simulink library "Lib_Turbo_Compressor_TMATS"  (R2012b)
settings: Solver=ode45  StartTime=0.0  StopTime=10.0  RelTol=1e-3
Description:
  | Thomas Modules
settings Model: Creator=jwchapm2  LastModifiedBy=jwchapm2

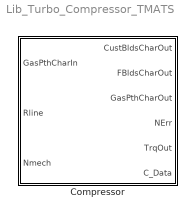
== system Lib_Turbo_Compressor_TMATS ==
  Compressor : Subsystem  mask(T-MATS: Compressor Library Block){X_C_RlineVec_M=[1.000 3.000 ], Y_C_NcVec_M=[0.500  0.900  1.050], T_C_Map_WcArray_M=[0 0; 0 0; 0 0], T_C_Map_PRArray_M=[0 0; 0 0; 0 0], T_C_Map_EffArray_M=[0 0; 0 0; 0 0], s_C_Nc_M=0.0001, s_C_Wc_M=0.4953, s_C_PR_M=0.8636, s_C_Eff_M=0.9977, CBLDEN_M=off, C_CBD_M=0, C_CBFht_M=0.5, C_CBFPt_M=0.5, FBLDEN_M=off, C_FBD_M=0, C_BFht_M=0.5, C_BFPt_M=0.5, X_C_WcSurgeVec_M=[0 200], T_C_PRSurgeVec_M=[30 30], iDesign_M=off, NcDes_M=10000, EffDes_M=0.95, PRDes_M=20, RlineDes_M=2}
      mask prompts: X_C_RlineVec_M "X_C_RlineVec_M - Compressor Map Rline Vector (X-axis)(nx1)"; Y_C_NcVec_M "Y_C_NcVec_M - Compressor Map Corrected Speed Vector (Y-axis)(mx1)"; T_C_Map_WcArray_M "T_C_Map_WcArray_M - Compressor Map Flow Array (Wc = f(Nc, Rline))(mxn)"; T_C_Map_PRArray_M "T_C_Map_PRArray_M - Compressor Map Pressure Ratio Array (PR = f(Nc, Rline))(mxn)"; T_C_Map_EffArray_M "T_C_Map_EffArray_M - Compressor Map Efficiency Array (Eff = f(Nc, Rline)(mxn)"; s_C_Nc_M "s_C_Nc_M - Corrected Speed Scalar Constant (C_Nc)"; s_C_Wc_M "s_C_Wc_M - Flow Scalar Constant (C_Wc)"; s_C_PR_M "s_C_PR_M - Pressure Ratio Scalar Constant (C_PR)"; s_C_Eff_M "s_C_Eff_M - Efficiency Scalar Constant (C_Eff)"; CBLDEN_M "CBLDEN_M - Customer Bleed Enable [0 - off, 1 - on]"; C_CBD_M "C_CBD_M - Customer or flow based Bleed Demand[pps] (cbx1)"; C_CBFht_M "C_CBFht_M - Customer or flow based Bleed Fractional enthalpy[frac] (cbx1)"; C_CBFPt_M "C_CBFPt_M - Customer or flow based Bleed Fractional Total Pressure[frac] (cbx1)"; FBLDEN_M "FBLDEN_M - Customer Bleed Enable [0 - off, 1 - on]"; C_FBD_M "C_FBD_M - Fractional Bleed Demand[frac] (bx1)"; C_BFht_M "C_BFht_M - engine Bleed Fractional enthalpy[frac] (bx1)"; C_BFPt_M "C_BFPt_M - engine Bleed Fractional Total Pressure[frac] (bx1)"; X_C_WcSurgeVec_M "X_C_WcSurgeVec_M - compensated flow Surge vector (sx1)"; T_C_PRSurgeVec_M "T_C_PRSurgeVec_M - Surge Line Pressure Ratio vector (sx1)"; iDesign_M "iDesign_M - Calculate compressor map scalars based on design variables"; NcDes_M "NcDes_M - map Design Corrected Shaft Speed [rpm]"; EffDes_M "EffDes_M  - Design Efficiency [frac]"; PRDes_M "PRDes_M - Design Pressure Ratio [frac]"; RlineDes_M "RlineDes_M - map Design Rline"
      mask help: This block simulates the performance of a compressor using basic thermodynamic equations, properties, and table lookups.
      mask Help: web(which('Turbo_TMATS_Cmp.html'),'-helpbrowser')
      mask Callback CBLDEN_M: MSK_SEC_Enables_TMATS('CBLDEN_M',[11 12 13],'en')
      mask Callback FBLDEN_M: MSK_SEC_Enables_TMATS('FBLDEN_M',[15 16 17],'en')
      mask Callback iDesign_M:
      | MSK_SEC_Enables_TMATS('iDesign_M',[21 22 23 24],'en')
      | MSK_SEC_Enables_TMATS('iDesign_M',[6 7 8 9],'dis')

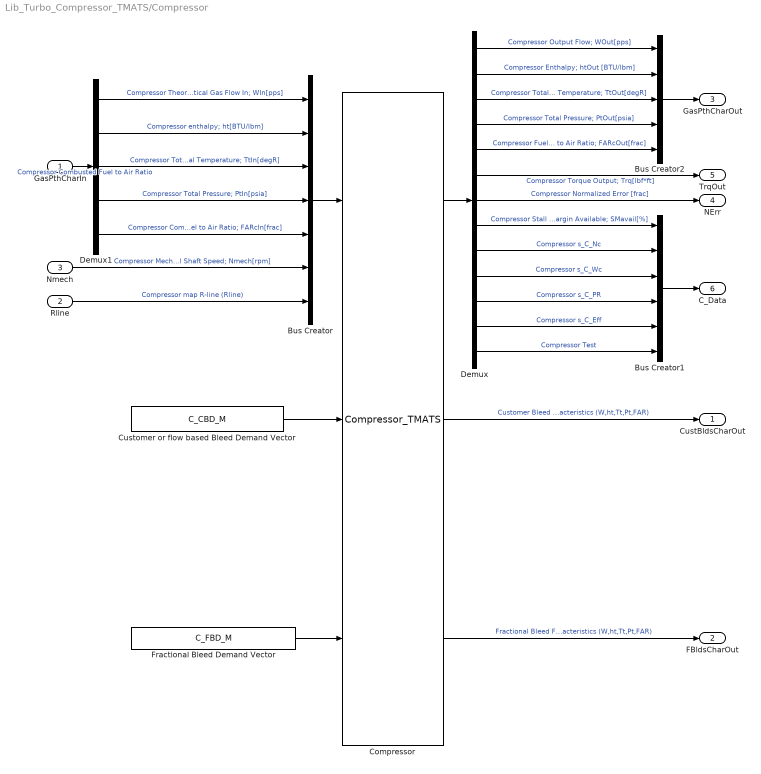
== system Lib_Turbo_Compressor_TMATS/Compressor ==
  GasPthCharIn : Inport
  Rline : Inport  Port=2
  Nmech : Inport  Port=3
  Bus Creator : BusCreator  Inputs=7
  Bus Creator1 : BusCreator  Inputs=6
  Bus Creator2 : BusCreator  Inputs=5
  Compressor : S-Function  FunctionName=Compressor_TMATS  Parameters="s_C_Nc_M, s_C_Wc_M, s_C_PR_M, s_C_Eff_M, Y_C_NcVec_M, X_C_RlineVec_M, T_C_Map_WcArray_M, T_C_Map_PRArray_M, T_C_Map_EffArray_M, C_CBFht_M, C_CBFPt_M,  C_BFht_M, C_BFPt_M, X_C_WcSurgeVec_M, T_C_PRSurgeVec_M, iDesign_M, NcDes_M, EffDes_M, PRDes_M, RlineDes_M, CBLDEN_M, FBLDEN_M, gcs"  EnableBusSupport=off
  Customer or flow based Bleed Demand Vector : Constant  Value=C_CBD_M
  Demux : Demux  Outputs=13
  Demux1 : Demux  Outputs=5
  Fractional Bleed Demand Vector : Constant  Value=C_FBD_M
  CustBldsCharOut : Outport
  FBldsCharOut : Outport  Port=2
  GasPthCharOut : Outport  Port=3
  NErr : Outport  Port=4
  TrqOut : Outport  Port=5
  C_Data : Outport  Port=6
  wires:
  Demux1/4 -> Bus Creator/4  "Compressor Total Pressure; PtIn[psia]"
  Nmech/1 -> Bus Creator/6  "Compressor Mechanical Shaft Speed; Nmech[rpm]"
  Demux/6 -> TrqOut/1  "Compressor Torque Output; Trq[lbf*ft]"
  Bus Creator/1 -> Compressor/1
  Demux/4 -> Bus Creator2/4  "Compressor Total Pressure; PtOut[psia]"
  Demux/3 -> Bus Creator2/3  "Compressor Total Temperature; TtOut[degR]"
  Demux/5 -> Bus Creator2/5  "Compressor Fuel to Air Ratio; FARcOut[frac]"
  Demux/1 -> Bus Creator2/1  "Compressor Output Flow; WOut[pps]"
  Compressor/1 -> Demux/1
  Demux1/3 -> Bus Creator/3  "Compressor Total Temperature; TtIn[degR]"
  Demux1/5 -> Bus Creator/5  "Compressor Combusted Fuel to Air Ratio; FARcIn[frac]"
  Rline/1 -> Bus Creator/7  "Compressor map R-line (Rline)"
  Demux/13 -> Bus Creator1/6  "Compressor Test"
  Demux/2 -> Bus Creator2/2  "Compressor Enthalpy; htOut [BTU/lbm]"
  Bus Creator2/1 -> GasPthCharOut/1
  GasPthCharIn/1 -> Demux1/1  "Compressor Combusted Fuel to Air Ratio"
  Demux1/1 -> Bus Creator/1  "Compressor Theoretical Gas Flow In; WIn[pps]"
  Demux/7 -> NErr/1  "Compressor Normalized Error [frac]"
  Customer or flow based Bleed Demand Vector/1 -> Compressor/2
  Fractional Bleed Demand Vector/1 -> Compressor/3
  Compressor/2 -> CustBldsCharOut/1  "Customer Bleed Characteristics (W,ht,Tt,Pt,FAR)"
  Compressor/3 -> FBldsCharOut/1  "Fractional Bleed Flow Characteristics (W,ht,Tt,Pt,FAR)"
  Demux1/2 -> Bus Creator/2  "Compressor enthalpy; ht[BTU/lbm]"
  Demux/8 -> Bus Creator1/1  "Compressor Stall Margin Available; SMavail[%]"
  Bus Creator1/1 -> C_Data/1
  Demux/9 -> Bus Creator1/2  "Compressor s_C_Nc"
  Demux/10 -> Bus Creator1/3  "Compressor s_C_Wc"
  Demux/11 -> Bus Creator1/4  "Compressor s_C_PR"
  Demux/12 -> Bus Creator1/5  "Compressor s_C_Eff"
